simulink model "StateMachine_Incorrect_paola"  (R2022b)
settings: Solver=VariableStepAuto  StartTime=0.0  StopTime=10.0  RelTol=1e-3
settings Model: Creator=jayerdi  LastModifiedBy=Pablo
settings OptimizationCC: ReuseModelBlockBuffer=on

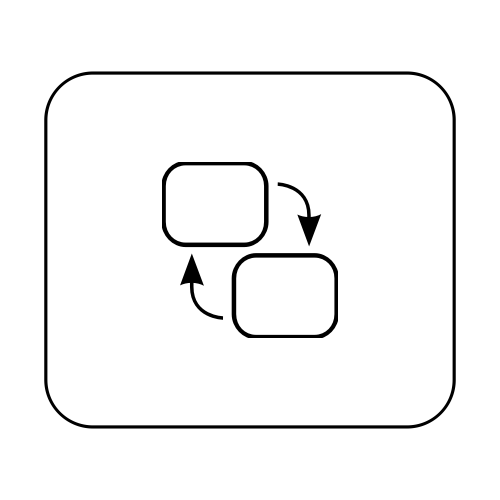
[thumbnail: Simulink's stored preview of the top-level diagram]
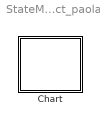
== system StateMachine_Incorrect_paola ==
  Chart : Stateflow chart  TreatAsAtomicUnit=on

== stateflow chart StateMachine_Incorrect_paola/Chart ==
  state State0
    v = 0;
    y = 0;
  state State1
    y = 1;
  state State2
    y = 3;
  state State3
    v = w;
  (default) -> State0
  State0 -> State1 [order 1] : [w > 3]
  State0 -> State2 [order 2] : [w > 5]
  State1 -> State3 : after(1,sec)
  State2 -> State3 : [z == 0]
